simulink model "APPL_PaFaultDetection"  (R2018b)
settings: configuration reference "CodeConfig_10_ms" (kept outside this file)
undefined symbols (not defined in the file): CAL_LockErrNoTime_30ms, CAL_ManualSwValid_90s, CAL_MotorHallInvalid_2s, CAL_MotorMaxRunTime_60s, CAL_MotorRelayErr_2s, CAL_MotorStall_750ms, D_DrSoftStopDef_B, D_DrSoftStopDef_F, D_DrSoftStopDef_H, D_DrSoftStopDef_L, D_Relay_DownBackFault, D_Relay_UpFrontFault, D_StallCurrent, enSeatMoveCmd, FALSE, TRUE
libraries: DareLib x91, simulink x2
(part 4 of 4)

== stateflow chart APPL_PaFaultDetection/LogicCtrl/AdheAndEffec/SwitchErrorDetection/GetDefTime/Chart ==
  (default) -> (junction 3)
  (junction 3) -> (junction 5)
  (junction 5) -> (junction 7) [order 1] : /* 设置比当前小 */
      | [DefTs < Ts]
  (junction 5) -> (junction 13) [order 2] : {OutTs = Ts - DefTs;}
  (junction 7) -> (junction 11) : {OutTs = 0xFFFFFFFF - DefTs;}
  (junction 11) -> (junction 13)
  (junction 13) -> (junction 17)
  data: DefTs input uint32; Ts input uint32; OutTs output uint32
